simulink model "real_estados_baltaslx"  (R2021a)
settings: Solver=VariableStepAuto  StartTime=0.0  StopTime=20  RelTol=1e-3
values from neighbouring files (symbols this model uses):
  A = [d3, d2, d1, y, du, u]    [PlantaEstable.m]    (also in real_estados_balta.m = [ -1.0135,  15.2396,       0,       0; test_chat.m = [ d3,    d2,    d1,    tita,    du,    u  ])
  Ad = eye(size(A)) + Ts * A    [observador_balta.m]    (also in observador_balta_2.m)
  Aoc = [A - Lc*C]    [estimacion_ecuaciones.m]    (also in observador_balta.m; observador_balta_2.m)
  B = [0; 0; 0; 131.4702]    [real_estados_balta.m]
  Bd = Ts * B    [observador_balta.m]    (also in observador_balta_2.m)
  C = [-6.2601, 94.1305, 0, 0]    [real_estados_balta.m]
  Cd = C    [observador_balta.m]    (also in observador_balta_2.m)
  Kc = acker(A,B,polyc)    [estimacion_ecuaciones.m]    (also in observador_balta.m; observador_balta_2.m)
  Lc = acker(A.',C.',polyec).'    [estimacion_ecuaciones.m]    (also in observador_balta.m; observador_balta_2.m)
settings Model: Creator=balta  LastModifiedBy=balta

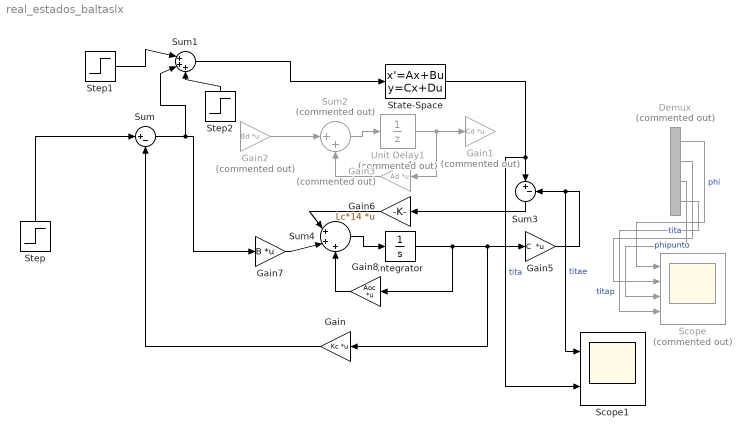
== system real_estados_baltaslx ==
  Demux : Demux  Commented=on
  Gain : Gain  Gain=Kc  Multiplication=Matrix(K*u)
  Gain1 : Gain  Commented=on  Gain=Cd  Multiplication=Matrix(K*u)
  Gain2 : Gain  Commented=on  Gain=Bd  Multiplication=Matrix(K*u)
  Gain3 : Gain  Commented=on  Gain=Ad  Multiplication=Matrix(K*u)
  Gain5 : Gain  Gain=C  Multiplication=Matrix(K*u)
  Gain6 : Gain  Gain=Lc*14  Multiplication=Matrix(K*u)
  Gain7 : Gain  Gain=B  Multiplication=Matrix(K*u)
  Gain8 : Gain  Gain=Aoc  Multiplication=Matrix(K*u)
  Integrator : Integrator
  Scope : Scope  Commented=on  NumInputPorts=4
  Scope1 : Scope  NumInputPorts=2
  State-Space : StateSpace  A=A  B=B  C=C  D=0  InitialCondition=0
  Step : Step  Time=0.1  After=0.01  SampleTime=0
  Step1 : Step  Time=0.1  After=10  SampleTime=0
  Step2 : Step  Time=0.5  After=-10  SampleTime=0
  Sum : Sum  Inputs=|+-
  Sum1 : Sum  Inputs=|+++
  Sum2 : Sum  Commented=on  Inputs=|++
  Sum3 : Sum  Inputs=|+-
  Sum4 : Sum  Inputs=|+++
  Unit Delay1 : UnitDelay  Commented=on  SampleTime=0.02  HasFrameUpgradeWarning=on
  wires:
  Gain2/1 -> Sum2/1
  Sum2/1 -> Unit Delay1/1
  Gain3/1 -> Sum2/2
  Gain6/1 -> Sum4/1
  Gain7/1 -> Sum4/2
  Gain8/1 -> Sum4/3
  Sum3/1 -> Gain6/1
  Sum4/1 -> Integrator/1
  Gain5/1 -> Scope1/1, Sum3/2  "titae"
  Unit Delay1/1 -> Gain3/1, Gain1/1
  Integrator/1 -> Gain8/1, Gain/1, Gain5/1
  Demux/1 -> Scope/1  "phi"
  Demux/2 -> Scope/2  "phipunto"
  Demux/3 -> Scope/3  "tita"
  Demux/4 -> Scope/4  "titap"
  State-Space/1 -> Scope1/2, Sum3/1  "tita"
  Gain/1 -> Sum/2
  Step/1 -> Sum/1
  Sum/1 -> Sum1/2, Gain7/1
  Sum1/1 -> State-Space/1
  Step1/1 -> Sum1/1
  Step2/1 -> Sum1/3
